simulink model "Inverted_Pendulum_2016b"  (Simulink 8.8)
settings: Solver=ode1  StartTime=0.0  StopTime=10  FixedStep=0.0001  RelTol=1e-3
values from neighbouring files (symbols this model uses):
  A_disc = sys_disc.A    [inverted_pend.m]
  B_disc = sys_disc.B    [inverted_pend.m]
  C_disc = sys_disc.C    [inverted_pend.m]
  D_disc = sys_disc.D    [inverted_pend.m]
  den_angle = [((M + m) * (I + m * L^2) - (m * L)^2), (b * (I + m * L^2)), - ((M + m) * m * g * L), - b * m * g * L]    [inverted_pend.m]
  den_angle_disc = cell2mat(angle_tf_disc.Denominator)    [inverted_pend.m]
  g = 9.8    [inverted_pend.m]
  m = 0.109    [inverted_pend.m]
  num_angle = [m * L, 0]    [inverted_pend.m]
  num_angle_disc = cell2mat(angle_tf_disc.Numerator)    [inverted_pend.m]
  R_kalman = [Measure_noise_position,              Measure_noise_speed,              Measure_noise_angle,              Measure_noise_angle_vel]    [inverted_pend.m]
  s = tf('s')    [inverted_pend.m]
  Time = 20    [inverted_pend.m]
  Time_step = 0.0001    [inverted_pend.m]
  Vk = [Measure_noise_position,              Measure_noise_speed,              Measure_noise_angle,              Measure_noise_angle_vel]    [inverted_pend.m]
  Wk = 0.0000001    (= 1e-07)    [inverted_pend.m]
undefined symbols (not defined in the file or in its folder): Discrete, K, X, Y, Z
libraries: sm_lib x18, nesl_utility x6, simulink x4, ctrlSharedLib x1
settings Model: Creator=gaoaidi  LastModifiedBy=15324
settings DataIOCC: LimitDataPoints=off  SaveFormat=Dataset  SignalLoggingSaveFormat=Dataset  ReturnWorkspaceOutputs=on
settings OptimizationCC: LifeSpan=auto
settings DebuggingCC: UnderspecifiedInitializationDetection=Simplified  MergeDetectMultiDrivingBlocksExec=error  FcnCallInpInsideContextMsg=error  StateNameClashWarn=none  SFUnexpectedBacktrackingDiag=error  SFNoUnconditionalDefaultTransitionDiag=error  SFExecutionAtInitializationDiag=warning
settings HardwareCC: ProdBitPerPointer=64  ProdBitPerSizeT=64  ProdBitPerPtrDiffT=64  ProdLargestAtomicFloat=Float  ProdIntDivRoundTo=Zero  ProdEndianess=LittleEndian  ProdWordSize=64  ProdHWDeviceType=Intel->x86-64 (Windows64)
settings ModelReferenceCC: PropagateSignalLabelsOutOfModel=on
settings SFSimCC: SimUseLocalCustomCode=on
settings RTWCC: RTWUseLocalCustomCode=on
settings GRTTargetCC: TargetLangStandard=C99 (ISO)  CombineOutputUpdateFcns=on  GRTInterface=off
settings ConfigComp: CovMetricSettings=dwe  CovSaveCumulativeToWorkspaceVar=off  CovSaveSingleToWorkspaceVar=off  CovExternalEMLEnable=on

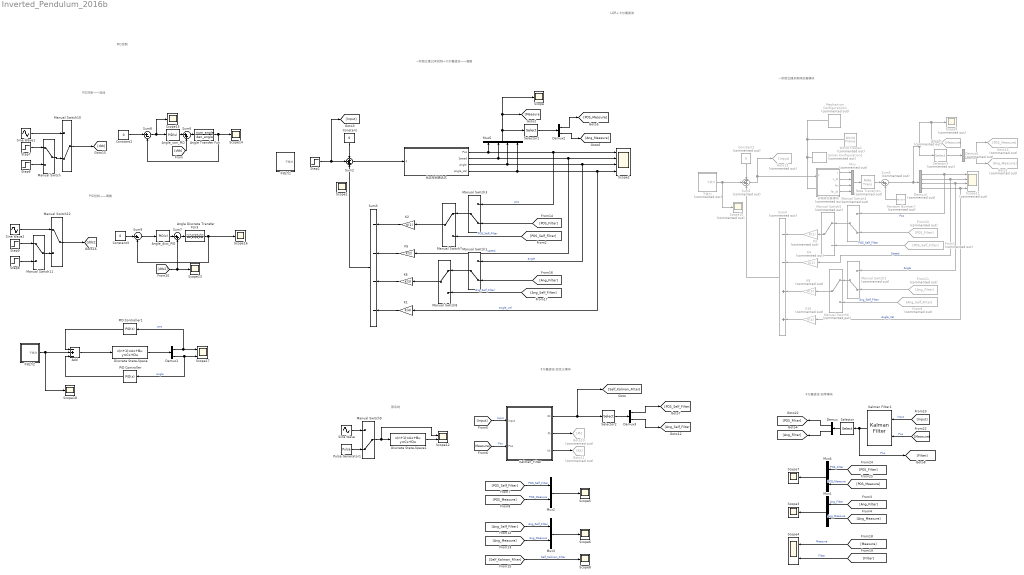
== system Inverted_Pendulum_2016b ==
  note: LQR+卡尔曼滤波
  note: 卡尔曼滤波-自带模块
  note: 一阶倒立摆LQR控制+卡尔曼滤波——离散
  note: 卡尔曼滤波-自定义模块
  note: 一阶倒立摆多刚体仿真模块
  note: 原系统
  note: PID控制——连续
  note: PID控制——离散
  note: PID控制
  Add : Sum  Inputs=-+-
  Angle Discrete Transfer Fcn3 : DiscreteTransferFcn  Numerator=num_angle_disc  Denominator=den_angle_disc
  Angle Transfer Fun : TransferFcn  Numerator=num_angle  Denominator=den_angle
  Angle_con_PID : simulink/Continuous/PID Controller  Controller=PID  Form=Parallel  TimeDomain=Continuous-time  SampleTime=0.01  IntegratorMethod=Forward Euler  ControllerParametersSource=internal  P=143.847551904  I=230.450310242486  D=16.9204342464564  N=2641.03068051249  UseFilter=on  InitialConditionSource=internal  InitialConditionForIntegrator=0  InitialConditionForFilter=0  DifferentiatorICPrevScaledInput=0  ExternalReset=none  TrackingMode=off  Kt=1  LimitOutput=off  UpperSaturationLimit=inf  LowerSaturationLimit=-inf  LinearizeAsGain=off  AntiWindupMode=none  Kb=1  POutMin=[]  POutMax=[]  IOutMin=[]  IOutMax=[]  DOutMin=[]  DOutMax=[]  NOutMin=[]  NOutMax=[]  SumOutMin=[]  SumOutMax=[]  SaturationOutMin=[]  SaturationOutMax=[]  PParamMin=[]  PParamMax=[]  IParamMin=[]  IParamMax=[]  DParamMin=[]  DParamMax=[]  NParamMin=[]  NParamMax=[]  KbParamMin=[]  KbParamMax=[]  KtParamMin=[]  KtParamMax=[]  KbOutMin=[]  KbOutMax=[]  KtOutMin=[]  KtOutMax=[]  IntegratorOutMin=[]  IntegratorOutMax=[]  FilterOutMin=[]  FilterOutMax=[]  SumI1OutMin=[]  SumI1OutMax=[]  SumI2OutMin=[]  SumI2OutMax=[]  SumI3OutMin=[]  SumI3OutMax=[]  SumDOutMin=[]  SumDOutMax=[]  DifferentiatorOutMin=[]  DifferentiatorOutMax=[]  IntegratorContinuousStateAttributes=''  IntegratorStateMustResolveToSignalObject=off  IntegratorRTWStateStorageClass=Auto  FilterContinuousStateAttributes=''  FilterStateMustResolveToSignalObject=off  FilterRTWStateStorageClass=Auto
  Angle_disc_PID : simulink/Continuous/PID Controller  Controller=PID  Form=Parallel  TimeDomain=Discrete-time  SampleTime=Time_step  IntegratorMethod=Forward Euler  ControllerParametersSource=internal  P=187.606066580867  I=461.512908325882  D=19.0655751892274  N=75.9625637841949  UseFilter=off  InitialConditionSource=internal  InitialConditionForIntegrator=0  InitialConditionForFilter=0  DifferentiatorICPrevScaledInput=0  ExternalReset=none  TrackingMode=off  Kt=1  LimitOutput=off  UpperSaturationLimit=inf  LowerSaturationLimit=-inf  LinearizeAsGain=off  AntiWindupMode=none  Kb=1  POutMin=[]  POutMax=[]  IOutMin=[]  IOutMax=[]  DOutMin=[]  DOutMax=[]  NOutMin=[]  NOutMax=[]  SumOutMin=[]  SumOutMax=[]  SaturationOutMin=[]  SaturationOutMax=[]  PParamMin=[]  PParamMax=[]  IParamMin=[]  IParamMax=[]  DParamMin=[]  DParamMax=[]  NParamMin=[]  NParamMax=[]  KbParamMin=[]  KbParamMax=[]  KtParamMin=[]  KtParamMax=[]  KbOutMin=[]  KbOutMax=[]  KtOutMin=[]  KtOutMax=[]  IntegratorOutMin=[]  IntegratorOutMax=[]  FilterOutMin=[]  FilterOutMax=[]  SumI1OutMin=[]  SumI1OutMax=[]  SumI2OutMin=[]  SumI2OutMax=[]  SumI3OutMin=[]  SumI3OutMax=[]  SumDOutMin=[]  SumDOutMax=[]  DifferentiatorOutMin=[]  DifferentiatorOutMax=[]  IntegratorContinuousStateAttributes=''  IntegratorStateMustResolveToSignalObject=off  IntegratorRTWStateStorageClass=Auto  FilterContinuousStateAttributes=''  FilterStateMustResolveToSignalObject=off  FilterRTWStateStorageClass=Auto
  Constant : Constant  Value=0  SampleTime=Time_step
  Constant1 : Constant  Commented=on  Value=0  SampleTime=Time_step
  Constant2 : Constant  Value=0
  Constant3 : Constant  Value=0  SampleTime=Time_step
  Demux{,1..3} (4 alike) : Demux  Outputs=2
  Demux4 : Demux  Commented=on
  Demux5 : Demux  Commented=on  Outputs=2
  Discrete State-Space : DiscreteStateSpace  A=A_disc  B=B_disc  C=[1 0 0 0;0 0 1 0]  D=[0 ; 0]  SampleTime=Time_step
  Discrete State-Space1 : DiscreteStateSpace  A=A_disc  B=B_disc  C=C_disc  D=D_disc  SampleTime=0.02
  From1 : From  Commented=on  GotoTag=POS_Self_Filter
  From10 : From  Commented=on  GotoTag=POS_Filter
  From11 : From  Commented=on  GotoTag=Ang_Filter
  From9 : From  Commented=on  GotoTag=Ang_Self_Filter
  Goto1 : Goto  Commented=on  GotoTag=Ang_Measure
  Goto10 : Goto  Commented=on  GotoTag=Pk
  Goto11 : Goto  Commented=on  GotoTag=Kk
  Goto13 : Goto  Commented=on  GotoTag=Input
  Goto14 : Goto  Commented=on  GotoTag=POS_Measure
  Goto9 : Goto  Commented=on  GotoTag=Measure
  K1 : Gain  Gain=K(4)
  K10 : Gain  Commented=on  Gain=K(4)
  K2 : Gain  Gain=K(1)
  K3 : Gain  Commented=on  Gain=K(1)
  K4 : Gain  Commented=on  Gain=K(2)
  K5 : Gain  Gain=K(2)
  K6 : Gain  Gain=K(3)
  K9 : Gain  Commented=on  Gain=K(3)
  Kalman Filter1 : ctrlSharedLib/Kalman Filter  TimeDomain=Discrete-Time  UseCurrentEstimator=on  ModelSource=Individual A, B, C, D matrices  ModelSourceVariable=ss(0.95,1,1,0,1)  A=A_disc  B=B_disc  C=C_disc  D=D_disc  NumberOfStates=1  NumberOfInputs=1  NumberOfOutputs=1  InitialEstimateSource=Dialog  X0=[0;0;0;0]  P0=10  UseK=off  UseGH=off  NumberOfProcessNoiseInputs=1  G=1  TimeInvariantG=on  H=0  TimeInvariantH=on  Q=Q_kalman  TimeInvariantQ=on  R=R_kalman  TimeInvariantR=on  N=0  TimeInvariantN=on  AddInputPort=on  AddEnablePort=off  OutputEstimatedY=off  OutputP=off  Ts=Time_step
  Kalman_Filter : Subsystem  mask{A=A_disc, B=B_disc, C=eye(4), D=[0;0;0;0], P0=0, X0=[0;0;0;0], Q=diag([0.00001 0 0.0001 0]), R=0.0001*eye(4)}
      mask prompts: A "ParameterA"; B "ParameterB"; C "ParameterC"; D "ParameterD"; P0 "ParameterP0"; X0 "ParameterX0"; Q "ParameterQ"; R "ParameterR"
      mask DialogControl BB Prompt: AA
  Manual Switch{,7..8,11..12} (5 alike) : ManualSwitch
  Manual Switch{1,3,9..10} (4 alike) : ManualSwitch  CurrentSetting=0
  Manual Switch2 : ManualSwitch  Commented=on  CurrentSetting=0
  Manual Switch4 : ManualSwitch  Commented=on  CurrentSetting=0
  Manual Switch5 : ManualSwitch  Commented=on
  Manual Switch6 : ManualSwitch  Commented=on
  Mechanism Configuration1 : sm_lib/Utilities/Mechanism Configuration  Commented=on  UniformGravity=Constant  GravityVector=[0 0 -9.80665]  GravityVectorUnits=m/s^2  LinearizationDelta=0.0001  JointModeTransitionNonlinearIterations=2
  Mux : Mux  Commented=on
  Mux{1..4} (4 alike) : Mux  Inputs=2
  Mux5 : Mux
  PID Controller : simulink/Continuous/PID Controller  Controller=PID  Form=Parallel  TimeDomain=Discrete-time  SampleTime=Time_step  IntegratorMethod=Forward Euler  ControllerParametersSource=internal  P=250  I=0  D=60  N=181.271400101852  UseFilter=on  InitialConditionSource=internal  InitialConditionForIntegrator=0  InitialConditionForFilter=0  DifferentiatorICPrevScaledInput=0  ExternalReset=none  TrackingMode=off  Kt=1  LimitOutput=off  UpperSaturationLimit=inf  LowerSaturationLimit=-inf  LinearizeAsGain=on  AntiWindupMode=none  Kb=1  POutMin=[]  POutMax=[]  IOutMin=[]  IOutMax=[]  DOutMin=[]  DOutMax=[]  NOutMin=[]  NOutMax=[]  SumOutMin=[]  SumOutMax=[]  SaturationOutMin=[]  SaturationOutMax=[]  PParamMin=[]  PParamMax=[]  IParamMin=[]  IParamMax=[]  DParamMin=[]  DParamMax=[]  NParamMin=[]  NParamMax=[]  KbParamMin=[]  KbParamMax=[]  KtParamMin=[]  KtParamMax=[]  KbOutMin=[]  KbOutMax=[]  KtOutMin=[]  KtOutMax=[]  IntegratorOutMin=[]  IntegratorOutMax=[]  FilterOutMin=[]  FilterOutMax=[]  SumI1OutMin=[]  SumI1OutMax=[]  SumI2OutMin=[]  SumI2OutMax=[]  SumI3OutMin=[]  SumI3OutMax=[]  SumDOutMin=[]  SumDOutMax=[]  DifferentiatorOutMin=[]  DifferentiatorOutMax=[]  IntegratorContinuousStateAttributes=''  IntegratorStateMustResolveToSignalObject=off  IntegratorRTWStateStorageClass=Auto  FilterContinuousStateAttributes=''  FilterStateMustResolveToSignalObject=off  FilterRTWStateStorageClass=Auto
  PID Controller1 : simulink/Continuous/PID Controller  Controller=PID  Form=Parallel  TimeDomain=Discrete-time  SampleTime=Time_step  IntegratorMethod=Forward Euler  ControllerParametersSource=internal  P=-90  I=-100  D=-70  N=276.52890372063  UseFilter=on  InitialConditionSource=internal  InitialConditionForIntegrator=0  InitialConditionForFilter=0  DifferentiatorICPrevScaledInput=0  ExternalReset=none  TrackingMode=off  Kt=1  LimitOutput=off  UpperSaturationLimit=inf  LowerSaturationLimit=-inf  LinearizeAsGain=on  AntiWindupMode=none  Kb=1  POutMin=[]  POutMax=[]  IOutMin=[]  IOutMax=[]  DOutMin=[]  DOutMax=[]  NOutMin=[]  NOutMax=[]  SumOutMin=[]  SumOutMax=[]  SaturationOutMin=[]  SaturationOutMax=[]  PParamMin=[]  PParamMax=[]  IParamMin=[]  IParamMax=[]  DParamMin=[]  DParamMax=[]  NParamMin=[]  NParamMax=[]  KbParamMin=[]  KbParamMax=[]  KtParamMin=[]  KtParamMax=[]  KbOutMin=[]  KbOutMax=[]  KtOutMin=[]  KtOutMax=[]  IntegratorOutMin=[]  IntegratorOutMax=[]  FilterOutMin=[]  FilterOutMax=[]  SumI1OutMin=[]  SumI1OutMax=[]  SumI2OutMin=[]  SumI2OutMax=[]  SumI3OutMin=[]  SumI3OutMax=[]  SumDOutMin=[]  SumDOutMax=[]  DifferentiatorOutMin=[]  DifferentiatorOutMax=[]  IntegratorContinuousStateAttributes=''  IntegratorStateMustResolveToSignalObject=off  IntegratorRTWStateStorageClass=Auto  FilterContinuousStateAttributes=''  FilterStateMustResolveToSignalObject=off  FilterRTWStateStorageClass=Auto
  Pulse Generator1 : DiscretePulseGenerator  PulseType=Time based  Period=15  PulseWidth=5  PhaseDelay=0.02
  Random Number2 : RandomNumber  Commented=on  Variance=0.0001  SampleTime=Time_step
  Rate Transition : RateTransition  Commented=on  OutPortSampleTime=Time_step
  Scope{,1,3,5..8,13..16,18} (12 alike) : Scope
  Scope10 : Scope  Commented=on
  Scope11 : Scope  Commented=on  NumInputPorts=4
  Scope12 : Scope  NumInputPorts=2
  Scope17 : Scope  NumInputPorts=2
  Scope2 : Scope  NumInputPorts=4
  Scope4 : Scope  NumInputPorts=2
  Scope9 : Scope  Commented=on
  Selector : Selector  InputPortWidth=4  IndexOptions=Index vector (dialog)  Indices=[1 3]  OutputSizes=1
  Selector1 : Selector  InputPortWidth=4  IndexOptions=Index vector (dialog)  Indices=[1 3]  OutputSizes=1
  Selector2 : Selector  InputPortWidth=4  IndexOptions=Index vector (dialog)  Indices=[1 3]  OutputSizes=1
  Selector3 : Selector  Commented=on  InputPortWidth=4  IndexOptions=Index vector (dialog)  Indices=[1 3]  OutputSizes=1
  Sine Wave : Sin  SampleTime=0.02
  Sine Wave1 : Sin  Frequency=2*pi  SampleTime=0
  Sine Wave2 : Sin  Frequency=2*pi  SampleTime=Time_step
  Solver Configuration1 : nesl_utility/Solver Configuration  Commented=on  PhysicalDomain=network_engine_domain  SubClassName=solver  LeftPortType=input  RightPortType=generic  Tones=[]  Harmonics=[]  SimulateNoise=off  Profile=off  UseLocalSampling=off  EnableSwitchedLinearOptims=on  FrequencyDomain=off  UseCCode=off  RelTol=0.001  AbsTol=1e-06  MinStep=1e-09  ToWorkspace=off  RevertToSquareIcSolve=off  NumHomotopyIterations=100  PhasorMode=off  PhasorModeNumHarmonics=1  ConsistencySolver=NEWTON_FTOL  IndexReductionMethod=DerivativeReplacement  DoDC=off  ResidualTolerance=1e-09  ConsistencyTolSource=GLOBAL  ConsistencyAbsTol=0.001  ConsistencyRelTol=0.001  ConsistencyTolFactor=0.001  UseLocalSolver=off  LocalSolverChoice=NE_BACKWARD_EULER_ADVANCER  ResolveIndetEquations=on  FunctionEvalNumThread=1  LocalSolverSampleTime=0.001  DoFixedCost=off  MaxNonlinIter=3  MaxModeIter=2  ComputeImpulses=off  ImpulseIterations=2  LinearAlgebra=auto  LinearAlgebraNumThread=0  EquationFormulation=NE_TIME_EF  DelaysMemoryBudget=1024  AutomaticFiltering=on  FilteringTimeConstant=0.001  PartitionStorageMethod=AS_NEEDED  PartitionMemoryBudget=1024  PartitionMethod=ROBUST  MultibodyUseLocalSolver=off  MultibodyLocalSolverChoice=ODE1  MultibodyLocalSolverSampleTime=0.001
  Step2 : Step  Before=20  After=0  SampleTime=Time_step
  Step6 : Step  Time=0.001  Before=1000  After=0  SampleTime=0
  Step7 : Step  Time=0  SampleTime=0
  Step8 : Step  Time=0.1  Before=10  After=0  SampleTime=Time_step
  Step9 : Step  Time=0  SampleTime=Time_step
  Sum1 : Sum  Commented=on  Inputs=+++
  Sum2 : Sum  Inputs=+++
  Sum3 : Sum  Inputs=----
  Sum4 : Sum  Commented=on  Inputs=--++
  Sum5 : Sum  Commented=on  Inputs=|++
  Sum6 : Sum  Inputs=|++
  Sum7 : Sum  Inputs=|++
  Sum8 : Sum  Inputs=|+-
  Sum9 : Sum  Inputs=|+-
  World Frame1 : sm_lib/Frames and Transforms/World Frame  Commented=on
  多刚体仿真模块 : Subsystem  Commented=on
  干扰力 : Subsystem  Commented=on  mask{Input=<empty>}
      mask prompts: Input "干扰力类型"
  干扰力1 : Subsystem  mask{Input=<empty>}
      mask prompts: Input "干扰力类型"
  干扰力2 : Subsystem  mask{Input=<empty>}
      mask prompts: Input "干扰力类型"
  状态空间表达式 : Subsystem  mask{A=A_disc, B=B_disc, C=C_disc, D=D_disc, Vk=Vk, Wk=Wk}
      mask prompts: Vk "测量噪声（vk）方差"; Wk "过程噪声（wk）方差（1*4）"
      mask DialogControl DescTextVar Prompt: 添加过程噪声及测量噪声的状态空间表达式
  wires:
  [POS_Measure] -> Mux4/2  "POS_Measure"
  [Measure] -> Kalman Filter1/2  "Pos"
  [Input] -> Kalman Filter1/1  "Input"
  Mux4/1 -> Scope7/1
  Kalman Filter1/1 -> [Filter], Selector/1  "Pos"
  Selector/1 -> Demux/1
  Demux/1 -> [POS_Filter]
  Demux/2 -> [Ang_Filter]
  Demux2/2 -> [Ang_Measure]
  Demux2/1 -> [POS_Measure]
  Selector1/1 -> Demux2/1
  [Ang_Measure] -> Mux1/2  "Ang_Measure"
  [Ang_Filter] -> Mux1/1  "Ang_Filter"
  Mux1/1 -> Scope3/1
  [POS_Filter] -> Mux4/1  "POS_Filter"
  Mux2/1 -> Scope5/1
  [POS_Measure] -> Mux2/2  "POS_Measure"
  [POS_Self_Filter] -> Mux2/1  "POS_Self_Filter"
  [Input] -> Kalman_Filter/1(input)  "Input"
  [Measure] -> Kalman_Filter/2(Pos)  "Pos"
  Kalman_Filter/1(Zk) -> Selector2/1, [Self_Kalman_Filter]
  Kalman_Filter/2(Pk) -> Goto10/1
  Kalman_Filter/3(Kk) -> Goto11/1
  Demux3/1 -> [POS_Self_Filter]
  Demux3/2 -> [Ang_Self_Filter]
  Selector2/1 -> Demux3/1
  [Ang_Self_Filter] -> Mux3/1  "Ang_Self_Filter"
  [Ang_Measure] -> Mux3/2  "Ang_Measure"
  Mux3/1 -> Scope6/1
  [Self_Kalman_Filter] -> Scope8/1  "Self_Kalman_Filter"
  Demux5/1 -> Goto14/1
  Demux5/2 -> Goto1/1
  Random Number2/1 -> Sum5/2
  K4/1 -> Sum4/2
  Sum5/1 -> Scope9/1, Goto9/1, Selector3/1, Demux4/1
  K10/1 -> Sum4/4
  Demux4/1 -> Manual Switch4/1, Scope11/1  "Pos"
  From10/1 -> Manual Switch4/2
  Demux4/4 -> K10/1, Scope11/4  "Angle_Vel"
  Selector3/1 -> Demux5/1
  Manual Switch6/1 -> K9/1
  Sum4/1 -> Sum1/3
  Demux4/2 -> K4/1, Scope11/2  "Speed"
  Demux4/3 -> Manual Switch2/1, Scope11/3  "Angle"
  多刚体仿真模块/1(x) -> Mux/1
  多刚体仿真模块/2(x_dt) -> Mux/2
  多刚体仿真模块/3(fai) -> Mux/3
  多刚体仿真模块/4(fai_dt) -> Mux/4
  Rate Transition/1 -> Sum5/1
  Sum1/1 -> 多刚体仿真模块/1(F), Goto13/1
  Mux/1 -> Rate Transition/1
  干扰力/1(干扰力) -> Sum1/2, Scope10/1
  Constant1/1 -> Sum1/1
  Constant/1 -> Sum2/1
  Manual Switch2/1 -> Manual Switch6/1
  Manual Switch4/1 -> Manual Switch5/1
  From1/1 -> Manual Switch5/2  "POS_Self_Filter"
  Manual Switch5/1 -> K3/1
  K3/1 -> Sum4/1
  K9/1 -> Sum4/3
  From9/1 -> Manual Switch6/2  "Ang_Self_Filter"
  From11/1 -> Manual Switch2/2
  Sum2/1 -> 状态空间表达式/1(F)
  状态空间表达式/4(Angle_Vel) -> Scope2/4, K1/1, Mux5/4  "angle_vel"
  Manual Switch8/1 -> K6/1
  [Ang_Filter] -> Manual Switch1/2
  K2/1 -> Sum3/1
  K6/1 -> Sum3/3
  [Ang_Self_Filter] -> Manual Switch8/2  "Ang_Self_Filter"
  [POS_Self_Filter] -> Manual Switch7/2  "POS_Self_Filter"
  Sum3/1 -> Sum2/3
  Manual Switch1/1 -> Manual Switch8/1
  K1/1 -> Sum3/4
  Manual Switch7/1 -> K2/1
  状态空间表达式/2(Speed) -> Scope2/2, K5/1, Mux5/2  "speed"
  状态空间表达式/3(Angle) -> Scope2/3, Manual Switch1/1, Mux5/3  "angle"
  [POS_Filter] -> Manual Switch3/2
  K5/1 -> Sum3/2
  状态空间表达式/1(Pos) -> Scope2/1, Manual Switch3/1, Mux5/1  "pos"
  Manual Switch3/1 -> Manual Switch7/1
  Mux5/1 -> Selector1/1, [Measure], Scope/1
  [Measure] -> Scope4/1  "Measure"
  [Filter] -> Scope4/2  "Filter"
  Pulse Generator1/1 -> Manual Switch9/2
  Sine Wave/1 -> Manual Switch9/1
  Manual Switch9/1 -> Scope12/1, Discrete State-Space1/1
  Discrete State-Space1/1 -> Scope12/2
  Manual Switch/1 -> Manual Switch10/2
  Sine Wave1/1 -> Manual Switch10/1
  Sum6/1 -> Angle Transfer Fun/1
  Constant3/1 -> Sum9/1
  Angle Discrete Transfer Fcn3/1 -> Scope16/1, Sum9/2
  [dtb2] -> Scope13/1, Sum7/2
  Manual Switch12/1 -> [dtb2]
  Sum9/1 -> Angle_disc_PID/1
  Manual Switch10/1 -> [dtb]
  Step9/1 -> Manual Switch11/1
  Manual Switch11/1 -> Manual Switch12/2
  Angle_con_PID/1 -> Sum6/1
  Step8/1 -> Manual Switch11/2
  Step7/1 -> Manual Switch/1
  Sum8/1 -> Scope15/1, Angle_con_PID/1
  Angle_disc_PID/1 -> Sum7/1
  Angle Transfer Fun/1 -> Scope14/1, Sum8/2
  Sine Wave2/1 -> Manual Switch12/1
  Sum7/1 -> Angle Discrete Transfer Fcn3/1
  Constant2/1 -> Sum8/1
  [dtb] -> Sum6/2
  Step6/1 -> Manual Switch/2
  Step2/1 -> [Input], Sum2/2
  Demux1/1 -> Scope17/1, PID Controller1/1  "pos"
  PID Controller1/1 -> Add/1
  Demux1/2 -> Scope17/2, PID Controller/1  "angle"
  Discrete State-Space/1 -> Demux1/1
  PID Controller/1 -> Add/3
  Add/1 -> Discrete State-Space/1
  干扰力2/1(干扰力) -> Add/2, Scope18/1
  connections:
  Mechanism Configuration1/RConn1 -- World Frame1/RConn1 -- Solver Configuration1/RConn1 -- 多刚体仿真模块/LConn1

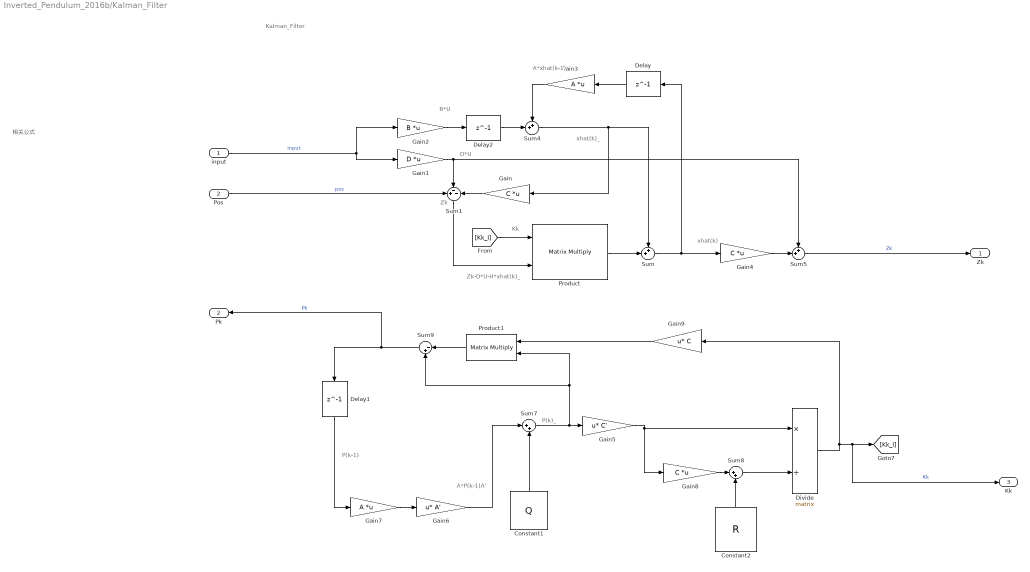
== system Inverted_Pendulum_2016b/Kalman_Filter ==
  note: 相关公式
  note: Kalman_Filter
  note: P(k-1)
  note: P(k)_
  note: A*P(k-1)A'
  note: A*xhat(k-1)
  note: xhat(k)
  note: Zk-D*U-H*xhat(k)_
  note: Kk
  note: Zk
  note: B*U
  note: D*U
  note: xhat(k)_
  input : Inport
  Pos : Inport  Port=2
  Constant1 : Constant  Value=Q  VectorParams1D=off
  Constant2 : Constant  Value=R  VectorParams1D=off
  Delay : Delay  DelayLength=1  InitialCondition=X0  UseCircularBuffer=on
  Delay1 : Delay  DelayLength=1  InitialCondition=P0  UseCircularBuffer=on
  Delay2 : Delay  DelayLength=1  InitialCondition=0  UseCircularBuffer=on
  Divide : Product  Inputs=*/  Multiplication=Matrix(*)
  Gain : Gain  Gain=C  Multiplication=Matrix(K*u)
  Gain1 : Gain  Gain=D  Multiplication=Matrix(K*u)
  Gain2 : Gain  Gain=B  Multiplication=Matrix(K*u)
  Gain3 : Gain  Gain=A  Multiplication=Matrix(K*u)
  Gain4 : Gain  Gain=C  Multiplication=Matrix(K*u)
  Gain5 : Gain  Gain=C'  Multiplication=Matrix(u*K)
  Gain6 : Gain  Gain=A'  Multiplication=Matrix(u*K)
  Gain7 : Gain  Gain=A  Multiplication=Matrix(K*u)
  Gain8 : Gain  Gain=C  Multiplication=Matrix(K*u)
  Gain9 : Gain  Gain=C  Multiplication=Matrix(u*K)
  Product : Product  Multiplication=Matrix(*)
  Product1 : Product  Multiplication=Matrix(*)
  Sum : Sum  Inputs=++|
  Sum1 : Sum  Inputs=+--
  Sum4 : Sum  Inputs=++|
  Sum5 : Sum  Inputs=++|
  Sum7 : Sum  Inputs=|++
  Sum8 : Sum  Inputs=|++
  Sum9 : Sum  Inputs=|-+
  Zk : Outport
  Pk : Outport  Port=2
  Kk : Outport  Port=3
  wires:
  Sum4/1 -> Sum/1, Gain/1
  Sum5/1 -> Zk/1  "Zk"
  Gain8/1 -> Sum8/1
  Product1/1 -> Sum9/1
  Gain/1 -> Sum1/3
  Sum/1 -> Gain4/1, Delay/1
  Gain5/1 -> Gain8/1, Divide/1
  Divide/1 -> Gain9/1, Kk/1, [Kk_I]  "Kk"
  [Kk_I] -> Product/1
  Sum9/1 -> Pk/1, Delay1/1  "Pk"
  Constant1/1 -> Sum7/2
  Gain1/1 -> Sum5/1, Sum1/2
  Delay2/1 -> Sum4/2
  Gain7/1 -> Gain6/1
  Sum1/1 -> Product/2
  input/1 -> Gain1/1, Gain2/1  "input"
  Sum8/1 -> Divide/2
  Sum7/1 -> Gain5/1, Product1/2, Sum9/2
  Gain6/1 -> Sum7/1
  Product/1 -> Sum/2
  Constant2/1 -> Sum8/2
  Pos/1 -> Sum1/1  "pos"
  Gain2/1 -> Delay2/1
  Gain4/1 -> Sum5/2
  Delay/1 -> Gain3/1
  Gain9/1 -> Product1/1
  Gain3/1 -> Sum4/1
  Delay1/1 -> Gain7/1

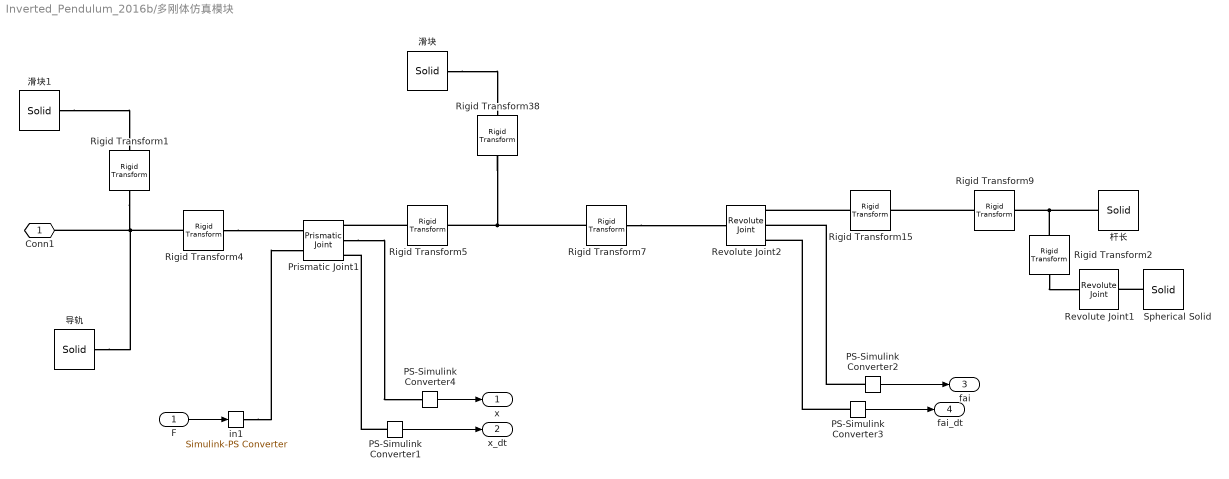
== system Inverted_Pendulum_2016b/多刚体仿真模块 ==
  F : Inport
  PS-Simulink Converter1 : nesl_utility/PS-Simulink Converter  PhysicalDomain=network_engine_domain  SubClassName=ps_output  LeftPortType=input  RightPortType=output  PseudoPeriodic=off  Frequencies=[]  VectorFormat=inherit  Unit=m/s  AffineConversion=off
  PS-Simulink Converter2 : nesl_utility/PS-Simulink Converter  PhysicalDomain=network_engine_domain  SubClassName=ps_output  LeftPortType=input  RightPortType=output  PseudoPeriodic=off  Frequencies=[]  VectorFormat=inherit  Unit=rad  AffineConversion=off
  PS-Simulink Converter3 : nesl_utility/PS-Simulink Converter  PhysicalDomain=network_engine_domain  SubClassName=ps_output  LeftPortType=input  RightPortType=output  PseudoPeriodic=off  Frequencies=[]  VectorFormat=inherit  Unit=rad/s  AffineConversion=off
  PS-Simulink Converter4 : nesl_utility/PS-Simulink Converter  PhysicalDomain=network_engine_domain  SubClassName=ps_output  LeftPortType=input  RightPortType=output  PseudoPeriodic=off  Frequencies=[]  VectorFormat=inherit  Unit=m  AffineConversion=off
  Prismatic Joint1 : sm_lib/Joints/Prismatic Joint  JointMode=Normal  SenseConstraintForce=off  SenseConstraintForceX=off  SenseConstraintForceY=off  SenseConstraintForceZ=off  SenseConstraintTorque=off  SenseConstraintTorqueX=off  SenseConstraintTorqueY=off  SenseConstraintTorqueZ=off  SenseTotalForce=off  SenseTotalForceX=off  SenseTotalForceY=off  SenseTotalForceZ=off  SenseTotalTorque=off  SenseTotalTorqueX=off  SenseTotalTorqueY=off  SenseTotalTorqueZ=off  CompositeWrenchDir=FollowerOnBase  CompositeWrenchFrame=BaseFrame  EquilibriumPosition=0  EquilibriumPositionUnits=m  SpringStiffness=0  SpringStiffnessUnits=N/m  DampingCoefficient=0  DampingCoefficientUnits=N/(m/s)  TorqueActuationMode=InputTorque  MotionActuationMode=ComputedMotion  SensePosition=on  SenseVelocity=on  SenseAcceleration=off  SenseTorqueForce=off  SenseLowerLimitTorqueForce=off  SenseUpperLimitTorqueForce=off  LowerLimitSpecify=off  LowerLimitBound=-1  LowerLimitBoundUnits=m  LowerLimitStiffness=1e6  LowerLimitStiffnessUnits=N/m  LowerLimitDamping=1e3  LowerLimitDampingUnits=N/(m/s)  LowerLimitTransitionRegionWidth=1e-4  LowerLimitTransitionRegionWidthUnits=m  UpperLimitSpecify=off  UpperLimitBound=1  UpperLimitBoundUnits=m  UpperLimitStiffness=1e6  UpperLimitStiffnessUnits=N/m  UpperLimitDamping=1e3  UpperLimitDampingUnits=N/(m/s)  UpperLimitTransitionRegionWidth=1e-4  UpperLimitTransitionRegionWidthUnits=m  PositionTargetSpecify=off  PositionTargetPriority=High  PositionTargetValue=0  PositionTargetValueUnits=m  VelocityTargetSpecify=off  VelocityTargetPriority=High  VelocityTargetValue=0  VelocityTargetValueUnits=m/s
  Revolute Joint1 : sm_lib/Joints/Revolute Joint  JointMode=Normal  SenseConstraintForce=off  SenseConstraintForceX=off  SenseConstraintForceY=off  SenseConstraintForceZ=off  SenseConstraintTorque=off  SenseConstraintTorqueX=off  SenseConstraintTorqueY=off  SenseConstraintTorqueZ=off  SenseTotalForce=off  SenseTotalForceX=off  SenseTotalForceY=off  SenseTotalForceZ=off  SenseTotalTorque=off  SenseTotalTorqueX=off  SenseTotalTorqueY=off  SenseTotalTorqueZ=off  CompositeWrenchDir=FollowerOnBase  CompositeWrenchFrame=BaseFrame  EquilibriumPosition=0  EquilibriumPositionUnits=deg  SpringStiffness=0  SpringStiffnessUnits=N*m/deg  DampingCoefficient=0  DampingCoefficientUnits=N*m/(deg/s)  TorqueActuationMode=NoTorque  MotionActuationMode=ComputedMotion  SensePosition=off  SenseVelocity=off  SenseAcceleration=off  SenseTorqueForce=off  SenseLowerLimitTorqueForce=off  SenseUpperLimitTorqueForce=off  LowerLimitSpecify=off  LowerLimitBound=-90  LowerLimitBoundUnits=deg  LowerLimitStiffness=1e4  LowerLimitStiffnessUnits=N*m/deg  LowerLimitDamping=10  LowerLimitDampingUnits=N*m/(deg/s)  LowerLimitTransitionRegionWidth=0.1  LowerLimitTransitionRegionWidthUnits=deg  UpperLimitSpecify=off  UpperLimitBound=90  UpperLimitBoundUnits=deg  UpperLimitStiffness=1e4  UpperLimitStiffnessUnits=N*m/deg  UpperLimitDamping=10  UpperLimitDampingUnits=N*m/(deg/s)  UpperLimitTransitionRegionWidth=0.1  UpperLimitTransitionRegionWidthUnits=deg  PositionTargetSpecify=on  PositionTargetPriority=High  PositionTargetValue=10  PositionTargetValueUnits=deg  VelocityTargetSpecify=off  VelocityTargetPriority=High  VelocityTargetValue=0  VelocityTargetValueUnits=deg/s
  Revolute Joint2 : sm_lib/Joints/Revolute Joint  JointMode=Normal  SenseConstraintForce=off  SenseConstraintForceX=off  SenseConstraintForceY=off  SenseConstraintForceZ=off  SenseConstraintTorque=off  SenseConstraintTorqueX=off  SenseConstraintTorqueY=off  SenseConstraintTorqueZ=off  SenseTotalForce=off  SenseTotalForceX=off  SenseTotalForceY=off  SenseTotalForceZ=off  SenseTotalTorque=off  SenseTotalTorqueX=off  SenseTotalTorqueY=off  SenseTotalTorqueZ=off  CompositeWrenchDir=FollowerOnBase  CompositeWrenchFrame=BaseFrame  EquilibriumPosition=0  EquilibriumPositionUnits=deg  SpringStiffness=0  SpringStiffnessUnits=N*m/deg  DampingCoefficient=0  DampingCoefficientUnits=N*m/(deg/s)  TorqueActuationMode=NoTorque  MotionActuationMode=ComputedMotion  SensePosition=on  SenseVelocity=on  SenseAcceleration=off  SenseTorqueForce=off  SenseLowerLimitTorqueForce=off  SenseUpperLimitTorqueForce=off  LowerLimitSpecify=off  LowerLimitBound=-90  LowerLimitBoundUnits=deg  LowerLimitStiffness=1e4  LowerLimitStiffnessUnits=N*m/deg  LowerLimitDamping=10  LowerLimitDampingUnits=N*m/(deg/s)  LowerLimitTransitionRegionWidth=0.1  LowerLimitTransitionRegionWidthUnits=deg  UpperLimitSpecify=off  UpperLimitBound=90  UpperLimitBoundUnits=deg  UpperLimitStiffness=1e4  UpperLimitStiffnessUnits=N*m/deg  UpperLimitDamping=10  UpperLimitDampingUnits=N*m/(deg/s)  UpperLimitTransitionRegionWidth=0.1  UpperLimitTransitionRegionWidthUnits=deg  PositionTargetSpecify=on  PositionTargetPriority=High  PositionTargetValue=10  PositionTargetValueUnits=deg  VelocityTargetSpecify=off  VelocityTargetPriority=High  VelocityTargetValue=0  VelocityTargetValueUnits=deg/s
  Rigid Transform1 : sm_lib/Frames and Transforms/Rigid Transform  TranslationMethod=None  TranslationStandardOffset=0  TranslationStandardOffsetUnits=m  TranslationStandardAxis=+Z  TranslationCartesianOffset=[0 0 0]  TranslationCartesianOffsetUnits=m  TranslationROffset=0  TranslationROffsetUnits=m  TranslationZOffset=0  TranslationZOffsetUnits=m  TranslationThetaOffset=0  TranslationThetaOffsetUnits=deg  RotationMethod=StandardAxis  RotationAngleUnits=deg  RotationStandardAxis=+Y  RotationAngle=90  RotationArbitraryAxis=[0 0 1]  FollAlignAxisA=+X  BaseAlignAxisA=+Y  FollAlignAxisB=+Y  BaseAlignAxisB=+Z  RotationSequenceAxes=FollowerAxes  RotationSequence=XYX  RotationSequenceAngles=[0 0 0]  RotationSequenceAnglesUnits=deg  RotationMatrix=[1 0 0; 0 1 0; 0 0 1]  Quaternion=[1 0 0 0]
  Rigid Transform15 : sm_lib/Frames and Transforms/Rigid Transform  TranslationMethod=None  TranslationStandardOffset=0  TranslationStandardOffsetUnits=m  TranslationStandardAxis=+Z  TranslationCartesianOffset=[0 0 0]  TranslationCartesianOffsetUnits=m  TranslationROffset=0  TranslationROffsetUnits=m  TranslationZOffset=0  TranslationZOffsetUnits=m  TranslationThetaOffset=0  TranslationThetaOffsetUnits=deg  RotationMethod=StandardAxis  RotationAngleUnits=deg  RotationStandardAxis=+X  RotationAngle=90  RotationArbitraryAxis=[0 0 1]  FollAlignAxisA=+X  BaseAlignAxisA=+Y  FollAlignAxisB=+Y  BaseAlignAxisB=+Z  RotationSequenceAxes=FollowerAxes  RotationSequence=XYX  RotationSequenceAngles=[0 0 0]  RotationSequenceAnglesUnits=deg  RotationMatrix=[1 0 0; 0 1 0; 0 0 1]  Quaternion=[1 0 0 0]
  Rigid Transform2 : sm_lib/Frames and Transforms/Rigid Transform  TranslationMethod=StandardAxis  TranslationStandardOffset=27  TranslationStandardOffsetUnits=cm  TranslationStandardAxis=+Z  TranslationCartesianOffset=[0 0 0]  TranslationCartesianOffsetUnits=cm  TranslationROffset=0  TranslationROffsetUnits=m  TranslationZOffset=0  TranslationZOffsetUnits=m  TranslationThetaOffset=0  TranslationThetaOffsetUnits=deg  RotationMethod=None  RotationAngleUnits=deg  RotationStandardAxis=+X  RotationAngle=90  RotationArbitraryAxis=[0 0 1]  FollAlignAxisA=+X  BaseAlignAxisA=+Y  FollAlignAxisB=+Y  BaseAlignAxisB=+Z  RotationSequenceAxes=FollowerAxes  RotationSequence=XYX  RotationSequenceAngles=[0 0 0]  RotationSequenceAnglesUnits=deg  RotationMatrix=[1 0 0; 0 1 0; 0 0 1]  Quaternion=[1 0 0 0]
  Rigid Transform38 : sm_lib/Frames and Transforms/Rigid Transform  TranslationMethod=None  TranslationStandardOffset=10  TranslationStandardOffsetUnits=cm  TranslationStandardAxis=-Y  TranslationCartesianOffset=[0 0 0]  TranslationCartesianOffsetUnits=cm  TranslationROffset=0  TranslationROffsetUnits=m  TranslationZOffset=0  TranslationZOffsetUnits=m  TranslationThetaOffset=0  TranslationThetaOffsetUnits=deg  RotationMethod=StandardAxis  RotationAngleUnits=deg  RotationStandardAxis=+X  RotationAngle=90  RotationArbitraryAxis=[0 0 1]  FollAlignAxisA=+X  BaseAlignAxisA=+Y  FollAlignAxisB=+Y  BaseAlignAxisB=+Z  RotationSequenceAxes=FollowerAxes  RotationSequence=XYX  RotationSequenceAngles=[0 0 0]  RotationSequenceAnglesUnits=deg  RotationMatrix=[1 0 0; 0 1 0; 0 0 1]  Quaternion=[1 0 0 0]
  Rigid Transform4 : sm_lib/Frames and Transforms/Rigid Transform  TranslationMethod=None  TranslationStandardOffset=0  TranslationStandardOffsetUnits=m  TranslationStandardAxis=+Z  TranslationCartesianOffset=[0 0 0]  TranslationCartesianOffsetUnits=m  TranslationROffset=0  TranslationROffsetUnits=m  TranslationZOffset=0  TranslationZOffsetUnits=m  TranslationThetaOffset=0  TranslationThetaOffsetUnits=deg  RotationMethod=StandardAxis  RotationAngleUnits=deg  RotationStandardAxis=+Y  RotationAngle=90  RotationArbitraryAxis=[0 0 1]  FollAlignAxisA=+X  BaseAlignAxisA=+Y  FollAlignAxisB=+Y  BaseAlignAxisB=+Z  RotationSequenceAxes=FollowerAxes  RotationSequence=XYX  RotationSequenceAngles=[0 0 0]  RotationSequenceAnglesUnits=deg  RotationMatrix=[1 0 0; 0 1 0; 0 0 1]  Quaternion=[1 0 0 0]
  Rigid Transform5 : sm_lib/Frames and Transforms/Rigid Transform  TranslationMethod=None  TranslationStandardOffset=0  TranslationStandardOffsetUnits=m  TranslationStandardAxis=+Z  TranslationCartesianOffset=[0 0 0]  TranslationCartesianOffsetUnits=m  TranslationROffset=0  TranslationROffsetUnits=m  TranslationZOffset=0  TranslationZOffsetUnits=m  TranslationThetaOffset=0  TranslationThetaOffsetUnits=deg  RotationMethod=StandardAxis  RotationAngleUnits=deg  RotationStandardAxis=+Y  RotationAngle=-90  RotationArbitraryAxis=[0 0 1]  FollAlignAxisA=+X  BaseAlignAxisA=+Y  FollAlignAxisB=+Y  BaseAlignAxisB=+Z  RotationSequenceAxes=FollowerAxes  RotationSequence=XYX  RotationSequenceAngles=[0 0 0]  RotationSequenceAnglesUnits=deg  RotationMatrix=[1 0 0; 0 1 0; 0 0 1]  Quaternion=[1 0 0 0]
  Rigid Transform7 : sm_lib/Frames and Transforms/Rigid Transform  TranslationMethod=None  TranslationStandardOffset=0  TranslationStandardOffsetUnits=m  TranslationStandardAxis=+Z  TranslationCartesianOffset=[0 0 0]  TranslationCartesianOffsetUnits=m  TranslationROffset=0  TranslationROffsetUnits=m  TranslationZOffset=0  TranslationZOffsetUnits=m  TranslationThetaOffset=0  TranslationThetaOffsetUnits=deg  RotationMethod=StandardAxis  RotationAngleUnits=deg  RotationStandardAxis=+X  RotationAngle=-90  RotationArbitraryAxis=[0 0 1]  FollAlignAxisA=+X  BaseAlignAxisA=+Y  FollAlignAxisB=+Y  BaseAlignAxisB=+Z  RotationSequenceAxes=FollowerAxes  RotationSequence=XYX  RotationSequenceAngles=[0 0 0]  RotationSequenceAnglesUnits=deg  RotationMatrix=[1 0 0; 0 1 0; 0 0 1]  Quaternion=[1 0 0 0]
  Rigid Transform9 : sm_lib/Frames and Transforms/Rigid Transform  TranslationMethod=StandardAxis  TranslationStandardOffset=25  TranslationStandardOffsetUnits=cm  TranslationStandardAxis=+Z  TranslationCartesianOffset=[0 0 0]  TranslationCartesianOffsetUnits=cm  TranslationROffset=0  TranslationROffsetUnits=m  TranslationZOffset=0  TranslationZOffsetUnits=m  TranslationThetaOffset=0  TranslationThetaOffsetUnits=deg  RotationMethod=None  RotationAngleUnits=deg  RotationStandardAxis=+X  RotationAngle=90  RotationArbitraryAxis=[0 0 1]  FollAlignAxisA=+X  BaseAlignAxisA=+Y  FollAlignAxisB=+Y  BaseAlignAxisB=+Z  RotationSequenceAxes=FollowerAxes  RotationSequence=XYX  RotationSequenceAngles=[0 0 0]  RotationSequenceAnglesUnits=deg  RotationMatrix=[1 0 0; 0 1 0; 0 0 1]  Quaternion=[1 0 0 0]
  Spherical Solid : sm_lib/Body Elements/Solid  GraphicAmbientColor=[0.15 0.15 0.15 1.0]  BasedOnType=Density  CenterOfMass=[0 0 0]  CenterOfMassUnits=m  GraphicDiffuseColor=[0.5 0.8 0.5]  Density=1  DensityUnits=kg/m^3  DoExposeReferenceFrame=on  GraphicEmissiveColor=[0.0 0.0 0.0 1.0]  ExportEntireGeometry=off  SerializedExposedGeometries=<exposedGeometries/>  SerializedFrames=<Frames/>  MarkerShape=Sphere  MarkerSize=10  GraphicType=FromGeometry  InertiaType=CalculateFromGeometry  Mass=1  MassUnits=kg  MomentsOfInertia=[1 1 1]  MomentsOfInertiaUnits=kg*m^2  GraphicOpacity=1.0  ProductsOfInertia=[0 0 0]  ProductsOfInertiaUnits=kg*m^2  GraphicShininess=75  GraphicSpecularColor=[0.5 0.5 0.5 1.0]  SphereRadius=3.5  SphereRadiusUnits=cm  GraphicVisPropType=SimpleVisualProperties
  in1 : nesl_utility/Simulink-PS Converter  PhysicalDomain=network_engine_domain  SubClassName=ps_input  LeftPortType=input  RightPortType=output  PseudoPeriodic=off  Frequencies=[]  NoiseDistribution=none  NoiseParameters=[]  Unit=1  AffineConversion=off  FilteringAndDerivatives=provide  SimscapeFilterOrder=1  InputFilterTimeConstant=0.001  UdotUserProvided=0
  导轨 : sm_lib/Body Elements/Solid  GraphicAmbientColor=[0.15 0.15 0.15 1.0]  BasedOnType=Density  BrickDimensions=[150 5 5]  BrickDimensionsUnits=cm  CenterOfMass=[0 0 0]  CenterOfMassUnits=m  GraphicDiffuseColor=[0 0 0]  Density=0.1  DensityUnits=g/cm^3  DoExposeReferenceFrame=on  GraphicEmissiveColor=[0.0 0.0 0.0 1.0]  ExportEntireGeometry=off  SerializedFrames=<Frames/>  MarkerShape=Sphere  MarkerSize=10  GraphicType=FromGeometry  InertiaType=CalculateFromGeometry  Mass=1  MassUnits=kg  MomentsOfInertia=[1 1 1]  MomentsOfInertiaUnits=kg*m^2  GraphicOpacity=1.0  ProductsOfInertia=[0 0 0]  ProductsOfInertiaUnits=kg*m^2  GraphicShininess=75  GraphicSpecularColor=[0.5 0.5 0.5 1.0]  GraphicVisPropType=SimpleVisualProperties
  杆长 : sm_lib/Body Elements/Solid  GraphicAmbientColor=[0.15 0.15 0.15 1.0]  BasedOnType=Density  BrickDimensions="[5 5  50]"  BrickDimensionsUnits=cm  CenterOfMass=[0 0 0]  CenterOfMassUnits=m  GraphicDiffuseColor=[0.8 0.5 0.1]  Density=0.1  DensityUnits=g/cm^3  DoExposeReferenceFrame=on  GraphicEmissiveColor=[0.0 0.0 0.0 1.0]  ExportEntireGeometry=off  SerializedFrames=<Frames/>  MarkerShape=Sphere  MarkerSize=10  GraphicType=FromGeometry  InertiaType=CalculateFromGeometry  Mass=1  MassUnits=kg  MomentsOfInertia=[1 1 1]  MomentsOfInertiaUnits=kg*m^2  GraphicOpacity=1.0  ProductsOfInertia=[0 0 0]  ProductsOfInertiaUnits=kg*m^2  GraphicShininess=75  GraphicSpecularColor=[0.5 0.5 0.5 1.0]  GraphicVisPropType=SimpleVisualProperties
  滑块 : sm_lib/Body Elements/Solid  GraphicAmbientColor=[0.15 0.15 0.15 1.0]  BasedOnType=Density  BrickDimensions=[10 10 10]  BrickDimensionsUnits=cm  CenterOfMass=[0 0 0]  CenterOfMassUnits=m  GraphicDiffuseColor=[0.1 0.1 0.8]  Density=0.1  DensityUnits=g/cm^3  DoExposeReferenceFrame=on  GraphicEmissiveColor=[0.0 0.0 0.0 1.0]  ExportEntireGeometry=off  SerializedFrames=<Frames/>  MarkerShape=Sphere  MarkerSize=10  GraphicType=FromGeometry  InertiaType=CalculateFromGeometry  Mass=1  MassUnits=kg  MomentsOfInertia=[1 1 1]  MomentsOfInertiaUnits=kg*m^2  GraphicOpacity=1.0  ProductsOfInertia=[0 0 0]  ProductsOfInertiaUnits=kg*m^2  GraphicShininess=75  GraphicSpecularColor=[0.5 0.5 0.5 1.0]  GraphicVisPropType=SimpleVisualProperties
  滑块1 : sm_lib/Body Elements/Solid  GraphicAmbientColor=[0.15 0.15 0.15 1.0]  BasedOnType=Density  BrickDimensions=[5 11 5]  BrickDimensionsUnits=cm  CenterOfMass=[0 0 0]  CenterOfMassUnits=m  GraphicDiffuseColor=[0.3 0.8 0.5]  Density=0.1  DensityUnits=g/cm^3  DoExposeReferenceFrame=on  GraphicEmissiveColor=[0.0 0.0 0.0 1.0]  ExportEntireGeometry=off  SerializedFrames=<Frames/>  MarkerShape=Sphere  MarkerSize=10  GraphicType=FromGeometry  InertiaType=CalculateFromGeometry  Mass=1  MassUnits=kg  MomentsOfInertia=[1 1 1]  MomentsOfInertiaUnits=kg*m^2  GraphicOpacity=1.0  ProductsOfInertia=[0 0 0]  ProductsOfInertiaUnits=kg*m^2  GraphicShininess=75  GraphicSpecularColor=[0.5 0.5 0.5 1.0]  GraphicVisPropType=SimpleVisualProperties
  Conn1 : PMIOPort  Side=Left
  x : Outport
  x_dt : Outport  Port=2
  fai : Outport  Port=3
  fai_dt : Outport  Port=4
  wires:
  F/1 -> in1/1
  PS-Simulink Converter1/1 -> x_dt/1
  PS-Simulink Converter3/1 -> fai_dt/1
  PS-Simulink Converter2/1 -> fai/1
  PS-Simulink Converter4/1 -> x/1
  connections:
  Rigid Transform9/LConn1 -- Rigid Transform15/RConn1
  in1/RConn1 -- Prismatic Joint1/LConn2
  Rigid Transform15/LConn1 -- Revolute Joint2/RConn1
  滑块/RConn1 -- Rigid Transform38/RConn1
  Rigid Transform7/RConn1 -- Revolute Joint2/LConn1
  Rigid Transform7/LConn1 -- Rigid Transform38/LConn1 -- Rigid Transform5/RConn1
  杆长/RConn1 -- Rigid Transform2/LConn1 -- Rigid Transform9/RConn1
  PS-Simulink Converter3/LConn1 -- Revolute Joint2/RConn3
  Rigid Transform5/LConn1 -- Prismatic Joint1/RConn1
  Rigid Transform4/RConn1 -- Prismatic Joint1/LConn1
  PS-Simulink Converter2/LConn1 -- Revolute Joint2/RConn2
  Rigid Transform4/LConn1 -- Conn1/RConn1 -- Rigid Transform1/RConn1 -- 导轨/RConn1
  PS-Simulink Converter1/LConn1 -- Prismatic Joint1/RConn3
  Prismatic Joint1/RConn2 -- PS-Simulink Converter4/LConn1
  滑块1/RConn1 -- Rigid Transform1/LConn1
  Spherical Solid/RConn1 -- Revolute Joint1/RConn1
  Rigid Transform2/RConn1 -- Revolute Joint1/LConn1

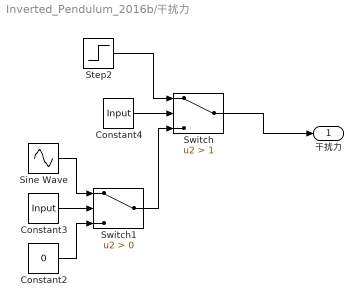
== system Inverted_Pendulum_2016b/干扰力 ==
  Constant2 : Constant  Value=0
  Constant3 : Constant  Value=Input
  Constant4 : Constant  Value=Input
  Sine Wave : Sin  SampleTime=Time_step
  Step2 : Step  Before=20  After=0  SampleTime=Time_step
  Switch : Switch  Criteria=u2 > Threshold  Threshold=1
  Switch1 : Switch  Criteria=u2 > Threshold
  干扰力 : Outport
  wires:
  Constant4/1 -> Switch/2
  Constant2/1 -> Switch1/3
  Switch/1 -> 干扰力/1
  Constant3/1 -> Switch1/2
  Switch1/1 -> Switch/3
  Sine Wave/1 -> Switch1/1
  Step2/1 -> Switch/1

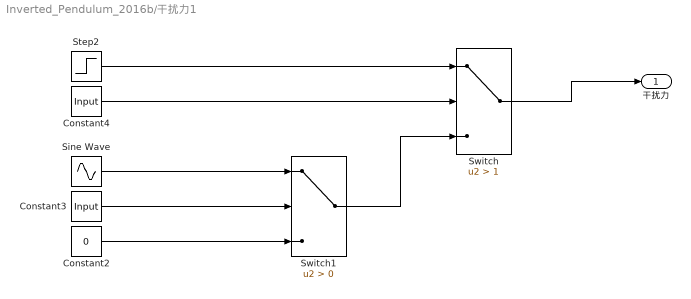
== system Inverted_Pendulum_2016b/干扰力1 ==
  Constant2 : Constant  Value=0
  Constant3 : Constant  Value=Input
  Constant4 : Constant  Value=Input
  Sine Wave : Sin  Amplitude=0.5  SampleTime=Time_step
  Step2 : Step  Before=20  After=0  SampleTime=Time_step
  Switch : Switch  Criteria=u2 > Threshold  Threshold=1
  Switch1 : Switch  Criteria=u2 > Threshold
  干扰力 : Outport
  wires:
  Constant4/1 -> Switch/2
  Constant2/1 -> Switch1/3
  Switch/1 -> 干扰力/1
  Constant3/1 -> Switch1/2
  Switch1/1 -> Switch/3
  Sine Wave/1 -> Switch1/1
  Step2/1 -> Switch/1

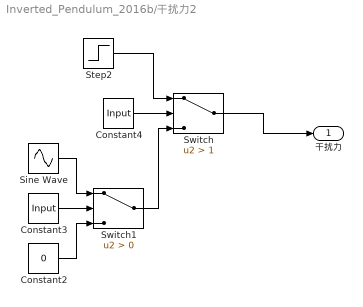
== system Inverted_Pendulum_2016b/干扰力2 ==
  Constant2 : Constant  Value=0
  Constant3 : Constant  Value=Input
  Constant4 : Constant  Value=Input
  Sine Wave : Sin  SampleTime=Time_step
  Step2 : Step  Before=2  After=0  SampleTime=Time_step
  Switch : Switch  Criteria=u2 > Threshold  Threshold=1
  Switch1 : Switch  Criteria=u2 > Threshold
  干扰力 : Outport
  wires:
  Constant4/1 -> Switch/2
  Constant2/1 -> Switch1/3
  Switch/1 -> 干扰力/1
  Constant3/1 -> Switch1/2
  Switch1/1 -> Switch/3
  Sine Wave/1 -> Switch1/1
  Step2/1 -> Switch/1

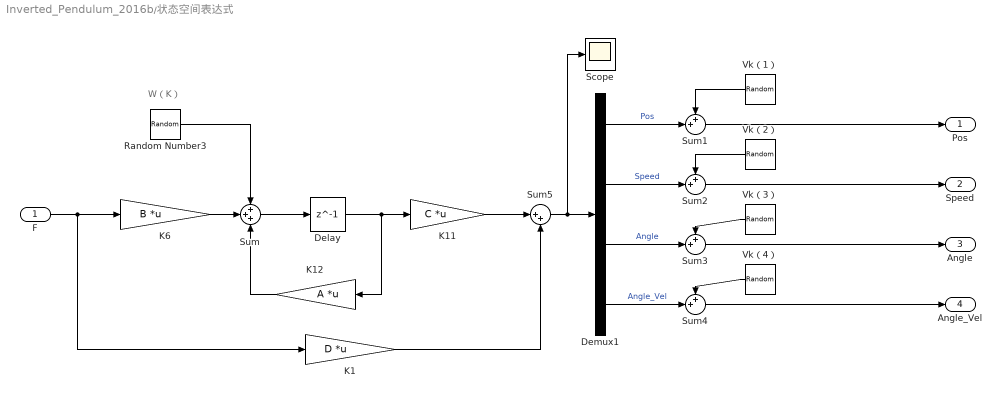
== system Inverted_Pendulum_2016b/状态空间表达式 ==
  note: W（K）
  F : Inport
  Delay : Delay  DelayLength=1
  Demux1 : Demux
  K1 : Gain  Gain=D  Multiplication=Matrix(K*u)
  K11 : Gain  Gain=C  Multiplication=Matrix(K*u)
  K12 : Gain  Gain=A  Multiplication=Matrix(K*u)
  K6 : Gain  Gain=B  Multiplication=Matrix(K*u)
  Random Number3 : RandomNumber  Variance=Wk  SampleTime=Time_step
  Scope : Scope
  Sum : Sum  Inputs=+++
  Sum{1..4} (4 alike) : Sum  Inputs=++|
  Sum5 : Sum  Inputs=|++
  Vk（1） : RandomNumber  Variance=Vk(1)  SampleTime=Time_step
  Vk（2） : RandomNumber  Variance=Vk(2)  SampleTime=Time_step
  Vk（3） : RandomNumber  Variance=Vk(3)  SampleTime=Time_step
  Vk（4） : RandomNumber  Variance=Vk(4)  SampleTime=Time_step
  Pos : Outport
  Speed : Outport  Port=2
  Angle : Outport  Port=3
  Angle_Vel : Outport  Port=4
  wires:
  Delay/1 -> K12/1, K11/1
  K12/1 -> Sum/3
  Random Number3/1 -> Sum/1
  K6/1 -> Sum/2
  Sum/1 -> Delay/1
  F/1 -> K1/1, K6/1
  Demux1/4 -> Sum4/2  "Angle_Vel"
  Sum1/1 -> Pos/1
  Demux1/3 -> Sum3/2  "Angle"
  Vk（1）/1 -> Sum1/1
  Demux1/1 -> Sum1/2  "Pos"
  Demux1/2 -> Sum2/2  "Speed"
  Vk（2）/1 -> Sum2/1
  Sum2/1 -> Speed/1
  Vk（3）/1 -> Sum3/1
  Sum3/1 -> Angle/1
  Vk（4）/1 -> Sum4/1
  Sum4/1 -> Angle_Vel/1
  K11/1 -> Sum5/1
  Sum5/1 -> Scope/1, Demux1/1
  K1/1 -> Sum5/2
